simulink model "modelSim_QuanserAero_AdaptiveV3"  (R2025b)
settings: Solver=FixedStepAuto  StartTime=0.0  StopTime=T  FixedStep=DAQ_time  MaxStep=0.01  RelTol=1e-3
values from neighbouring files (symbols this model uses):
  A_cmd = [Ap_cmd, Ay_cmd]    [runExperiment_QuanserAero_Hardware_AdaptiveV4_1DOF_pitch.m]    (also in runExperiment_QuanserAero_Hardware_AdaptiveV4_1DOF_yaw.m; runSim_QuanserAero_AdaptiveV3.m; run_QuanserAero_AdaptiveV3_SN.m)
  a_cmd_coeff = [ap_cmd_coeff,ay_cmd_coeff]    [runExperiment_QuanserAero_Hardware_AdaptiveV4_1DOF_pitch.m]    (also in runExperiment_QuanserAero_Hardware_AdaptiveV4_1DOF_yaw.m; runSim_QuanserAero_AdaptiveV3.m; run_QuanserAero_AdaptiveV3_SN.m)
  cmd_select = [1,0]    [runExperiment_QuanserAero_Hardware_AdaptiveV4_1DOF_pitch.m]    (also in runExperiment_QuanserAero_Hardware_AdaptiveV4_1DOF_yaw.m = [1,1]; runSim_QuanserAero_AdaptiveV3.m = [0,2]; run_QuanserAero_AdaptiveV3_SN.m = [0,2])
  control_gains = [lambda_p lambda_y ... (first row only)    [runExperiment_QuanserAero_Hardware_AdaptiveV4_1DOF_pitch.m]    (also in runExperiment_QuanserAero_Hardware_AdaptiveV4_1DOF_yaw.m; runSim_QuanserAero_AdaptiveV3.m; run_QuanserAero_AdaptiveV3_SN.m)
  gamma_p = [gamma0_p;gamma1_p;gamma2_p;gamma3_p;gamma4_p]    [runExperiment_QuanserAero_Hardware_AdaptiveV4_1DOF_pitch.m]    (also in runExperiment_QuanserAero_Hardware_AdaptiveV4_1DOF_yaw.m; runSim_QuanserAero_AdaptiveV3.m; run_QuanserAero_AdaptiveV3_SN.m)
  gamma_y = [gamma0_y;gamma1_y;gamma2_y;gamma3_y]    [runExperiment_QuanserAero_Hardware_AdaptiveV4_1DOF_pitch.m]    (also in runExperiment_QuanserAero_Hardware_AdaptiveV4_1DOF_yaw.m; runSim_QuanserAero_AdaptiveV3.m; run_QuanserAero_AdaptiveV3_SN.m)
  harmonic_cutoff_p = Tp_cmd*harmonic_cycles    (= 20)    [runExperiment_QuanserAero_Hardware_AdaptiveV4_1DOF_pitch.m]    (also in runExperiment_QuanserAero_Hardware_AdaptiveV4_1DOF_yaw.m; runSim_QuanserAero_AdaptiveV3.m; run_QuanserAero_AdaptiveV3_SN.m)
  harmonic_cutoff_y = Ty_cmd*harmonic_cycles    (= 20)    [runExperiment_QuanserAero_Hardware_AdaptiveV4_1DOF_pitch.m]    (also in runExperiment_QuanserAero_Hardware_AdaptiveV4_1DOF_yaw.m; runSim_QuanserAero_AdaptiveV3.m; run_QuanserAero_AdaptiveV3_SN.m = 40)
  paramsGuess_haaaa = [hp_hat hy_hat ... (first row only)    [runExperiment_QuanserAero_Hardware_AdaptiveV4_1DOF_pitch.m]    (also in runExperiment_QuanserAero_Hardware_AdaptiveV4_1DOF_yaw.m; runSim_QuanserAero_AdaptiveV3.m; run_QuanserAero_AdaptiveV3_SN.m)
  paramsTruth_haaaa = paramsGuess_haaaa.*paramsError_haaaa    [runSim_QuanserAero_AdaptiveV3.m]    (also in run_QuanserAero_AdaptiveV3_SN.m)
  T_cmd = [Tp_cmd, Ty_cmd]    [runExperiment_QuanserAero_Hardware_AdaptiveV4_1DOF_pitch.m]    (also in runExperiment_QuanserAero_Hardware_AdaptiveV4_1DOF_yaw.m; runSim_QuanserAero_AdaptiveV3.m; run_QuanserAero_AdaptiveV3_SN.m)
settings Model: Creator=ryanmathewson  LastModifiedBy=samue
settings DebuggingCC: UnconnectedInputMsg=warning  UnconnectedOutputMsg=warning  UnconnectedLineMsg=warning
settings ModelReferenceCC: EnableRefExpFcnMdlSchedulingChecks=on
settings RTWCC: GPUComputeCapability=3.5  DLArmComputeVersion=19.05

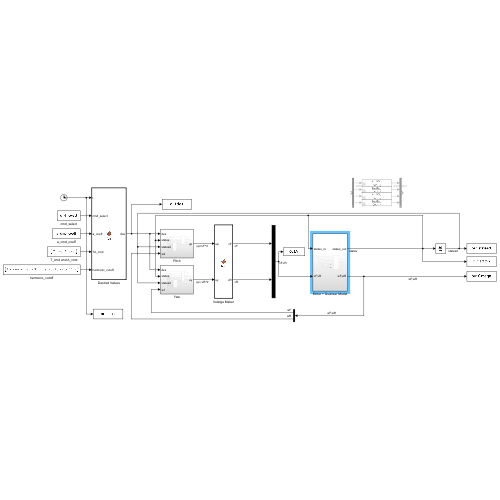
[thumbnail: Simulink's stored preview of the top-level diagram]
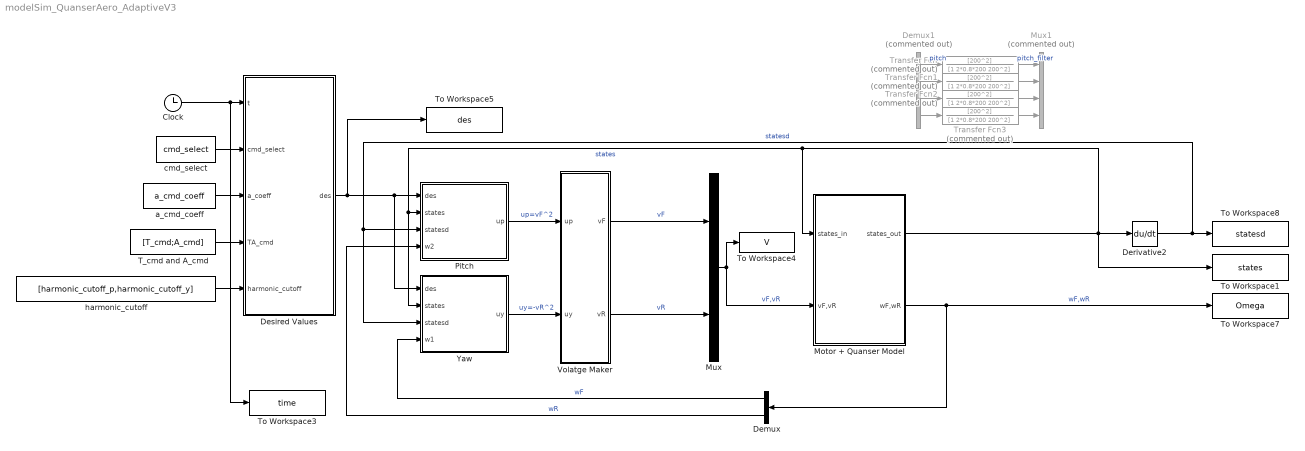
== system modelSim_QuanserAero_AdaptiveV3 ==
  Clock : Clock
  Demux : Demux  Outputs=2
  Demux1 : Demux  Commented=on
  Derivative2 : Derivative
  Desired Values : MATLAB Function  TreatAsAtomicUnit=on
  Motor + Quanser Model : Subsystem
  Mux : Mux  Inputs=2
  Mux1 : Mux  Commented=on
  Pitch : Subsystem
  T_cmd and A_cmd : Constant  Value=[T_cmd;A_cmd]
  To Workspace1 : ToWorkspace  VariableName=states  SampleTime=-1
  To Workspace3 : ToWorkspace  VariableName=time  SampleTime=-1
  To Workspace4 : ToWorkspace  VariableName=V  SampleTime=-1
  To Workspace5 : ToWorkspace  VariableName=des  SampleTime=-1
  To Workspace7 : ToWorkspace  VariableName=Omega  SampleTime=-1
  To Workspace8 : ToWorkspace  VariableName=statesd  SampleTime=-1
  Transfer Fcn{,1..3} (4 alike) : TransferFcn  Commented=on  Numerator=[200^2]  Denominator=[1 2*0.8*200 200^2]
  Volatge Maker : MATLAB Function  TreatAsAtomicUnit=on
  Yaw : Subsystem
  a_cmd_coeff : Constant  Value=a_cmd_coeff
  cmd_select : Constant  Value=cmd_select
  harmonic_cutoff : Constant  Value=[harmonic_cutoff_p,harmonic_cutoff_y]
  wires:
  Clock/1 -> To Workspace3/1, Desired Values/1(t)
  Desired Values/1(des) -> To Workspace5/1, Yaw/1(des), Pitch/1(des)
  Pitch/1(up) -> Volatge Maker/1(up)  "up=vF^2"
  Yaw/1(uy) -> Volatge Maker/2(uy)  "uy=-vR^2"
  Volatge Maker/1(vF) -> Mux/1  "vF"
  Derivative2/1 -> To Workspace8/1, Pitch/3(statesd), Yaw/3(statesd)  "statesd"
  Mux/1 -> Motor + Quanser Model/2(vF,vR), To Workspace4/1  "vF,vR"
  Volatge Maker/2(vR) -> Mux/2  "vR"
  Motor + Quanser Model/2(wF,wR) -> Demux/1, To Workspace7/1  "wF,wR"
  Demux/1 -> Yaw/4(w1)  "wF"
  Demux/2 -> Pitch/4(w2)  "wR"
  Motor + Quanser Model/1(states_out) -> Motor + Quanser Model/1(states_in), Pitch/2(states), Yaw/2(states), To Workspace1/1, Derivative2/1  "states"
  a_cmd_coeff/1 -> Desired Values/3(a_coeff)
  cmd_select/1 -> Desired Values/2(cmd_select)
  T_cmd and A_cmd/1 -> Desired Values/4(TA_cmd)
  harmonic_cutoff/1 -> Desired Values/5(harmonic_cutoff)
  Demux1/1 -> Transfer Fcn/1  "pitch"
  Demux1/3 -> Transfer Fcn2/1
  Demux1/2 -> Transfer Fcn1/1
  Demux1/4 -> Transfer Fcn3/1
  Transfer Fcn/1 -> Mux1/1  "pitch_filter"
  Transfer Fcn1/1 -> Mux1/2
  Transfer Fcn2/1 -> Mux1/3
  Transfer Fcn3/1 -> Mux1/4

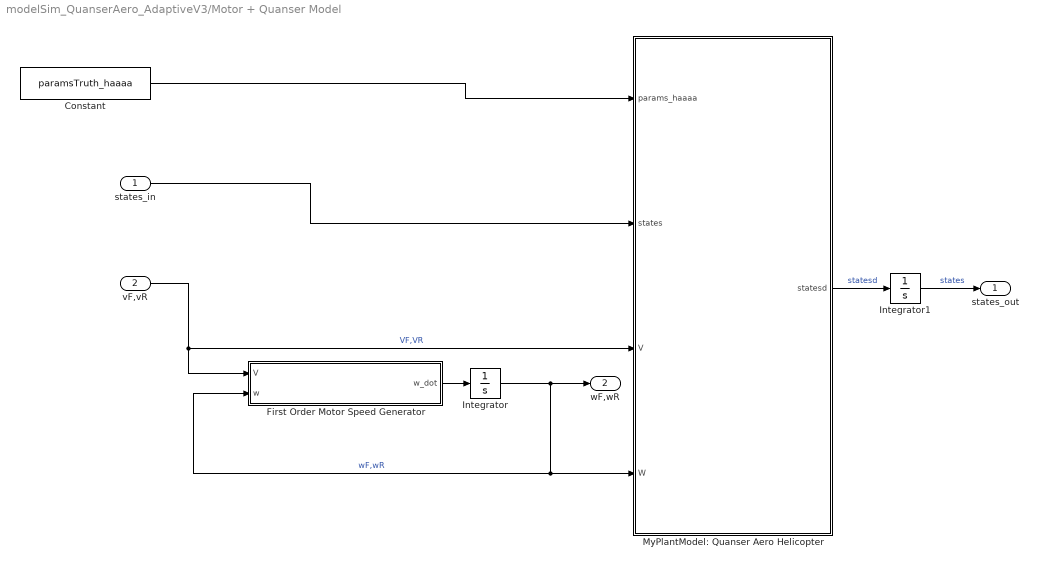
== system modelSim_QuanserAero_AdaptiveV3/Motor + Quanser Model ==
  states_in : Inport  PortDimensions=[4 1]
  vF,vR : Inport  Port=2  PortDimensions=[2 1]
  Constant : Constant  Value=paramsTruth_haaaa
  First Order Motor Speed Generator : MATLAB Function  TreatAsAtomicUnit=on
  Integrator : Integrator  InitialCondition=[0;0]
  Integrator1 : Integrator  InitialCondition=[0;0;0;0]
  MyPlantModel: Quanser Aero Helicopter : MATLAB Function  TreatAsAtomicUnit=on
  states_out : Outport  PortDimensions=[4 1]
  wF,wR : Outport  Port=2  PortDimensions=[2 1]
  wires:
  states_in/1 -> MyPlantModel: Quanser Aero Helicopter/2(states)
  vF,vR/1 -> First Order Motor Speed Generator/1(V), MyPlantModel: Quanser Aero Helicopter/3(V)  "VF,VR"
  MyPlantModel: Quanser Aero Helicopter/1(statesd) -> Integrator1/1  "statesd"
  First Order Motor Speed Generator/1(w_dot) -> Integrator/1
  Constant/1 -> MyPlantModel: Quanser Aero Helicopter/1(params_haaaa)
  Integrator1/1 -> states_out/1  "states"
  Integrator/1 -> First Order Motor Speed Generator/2(w), MyPlantModel: Quanser Aero Helicopter/4(W), wF,wR/1  "wF,wR"

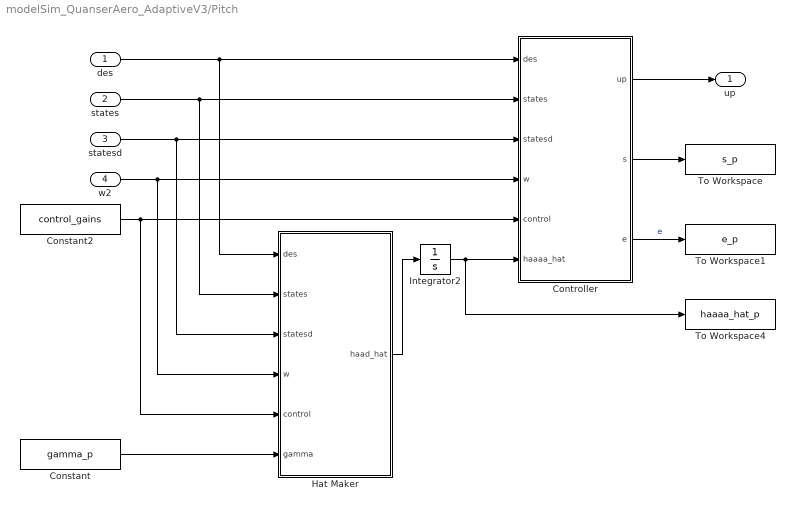
== system modelSim_QuanserAero_AdaptiveV3/Pitch ==
  des : Inport
  states : Inport  Port=2
  statesd : Inport  Port=3
  w2 : Inport  Port=4
  Constant : Constant  Value=gamma_p
  Constant2 : Constant  Value=control_gains
  Controller : MATLAB Function  TreatAsAtomicUnit=on
  Hat Maker : MATLAB Function  TreatAsAtomicUnit=on
  Integrator2 : Integrator  InitialCondition=paramsGuess_haaaa(:,1)
  To Workspace : ToWorkspace  VariableName=s_p  SampleTime=-1
  To Workspace1 : ToWorkspace  VariableName=e_p  SampleTime=-1
  To Workspace4 : ToWorkspace  VariableName=haaaa_hat_p  SampleTime=-1
  up : Outport
  wires:
  Integrator2/1 -> To Workspace4/1, Controller/6(haaaa_hat)
  Hat Maker/1(haad_hat) -> Integrator2/1
  Controller/1(up) -> up/1
  states/1 -> Hat Maker/2(states), Controller/2(states)
  Controller/2(s) -> To Workspace/1
  des/1 -> Hat Maker/1(des), Controller/1(des)
  statesd/1 -> Hat Maker/3(statesd), Controller/3(statesd)
  w2/1 -> Hat Maker/4(w), Controller/4(w)
  Constant2/1 -> Hat Maker/5(control), Controller/5(control)
  Constant/1 -> Hat Maker/6(gamma)
  Controller/3(e) -> To Workspace1/1  "e"

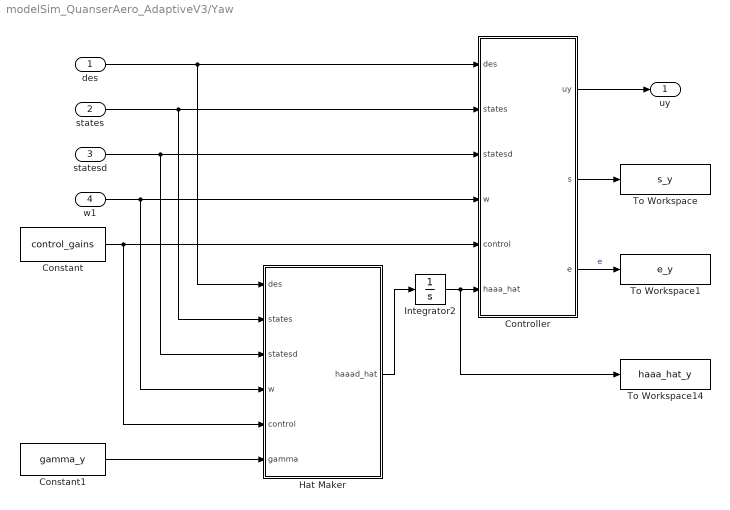
== system modelSim_QuanserAero_AdaptiveV3/Yaw ==
  des : Inport
  states : Inport  Port=2
  statesd : Inport  Port=3
  w1 : Inport  Port=4
  Constant : Constant  Value=control_gains
  Constant1 : Constant  Value=gamma_y
  Controller : MATLAB Function  TreatAsAtomicUnit=on
  Hat Maker : MATLAB Function  TreatAsAtomicUnit=on
  Integrator2 : Integrator  InitialCondition=paramsGuess_haaaa(1:4,2)
  To Workspace : ToWorkspace  VariableName=s_y  SampleTime=-1
  To Workspace1 : ToWorkspace  VariableName=e_y  SampleTime=-1
  To Workspace14 : ToWorkspace  VariableName=haaa_hat_y  SampleTime=-1
  uy : Outport
  wires:
  Integrator2/1 -> To Workspace14/1, Controller/6(haaa_hat)
  des/1 -> Controller/1(des), Hat Maker/1(des)
  Hat Maker/1(haaad_hat) -> Integrator2/1
  Controller/1(uy) -> uy/1
  Controller/2(s) -> To Workspace/1
  states/1 -> Controller/2(states), Hat Maker/2(states)
  statesd/1 -> Controller/3(statesd), Hat Maker/3(statesd)
  w1/1 -> Controller/4(w), Hat Maker/4(w)
  Controller/3(e) -> To Workspace1/1  "e"
  Constant/1 -> Controller/5(control), Hat Maker/5(control)
  Constant1/1 -> Hat Maker/6(gamma)

== matlab function modelSim_QuanserAero_AdaptiveV3/Yaw/Hat Maker ==
  data: des input; states input; haaad_hat output; statesd input; w input; control input; gamma input
function haaad_hat = fcn(des,states,statesd, w, control, gamma)
%% initialize outputs
haaad_hat = zeros(4,1);

%% separate input vectors
% desired variables
yaw_des = des(4,1);
yawd_des = des(5,1);
yawdd_des = des(6,1);
% state variables
r_yaw = states(3,1);
% state derivative variables
rd_yaw = statesd(3,1);
rdd_yaw = statesd(4,1);
% motor angular velocity
r_omega_f = w;
% controller gains
lambda = control(1,2);
D = control(2,2);
eta = control(3,2);
phi_para = control(4,2);
gamma_0 = gamma(1,1);
gamma_1 = gamma(2,1);
gamma_2 = gamma(3,1);
gamma_3 = gamma(4,1);

%% functions
e = r_yaw-yaw_des;
ed = rd_yaw-yawd_des;
yawdd_ref = -(-yawdd_des + lambda*ed) ; %2*lambda*ed + lambda^2*e;
s = ed + lambda*e;
ds = rdd_yaw - yawdd_ref;

%saturation function
% if s>phi_para
%   sat = 1;
% elseif (s>=-phi_para)&&(s<=phi_para)
%   sat = s/phi_para;
% else
%   sat = -1;
% end
if abs(s)>phi_para
    sat = sign(s);
else
    sat = s/phi_para;
end
s_delta = s - (phi_para * sat);

f1 = rd_yaw;
f2 = r_omega_f;
f3 = sign(r_omega_f)*r_omega_f^2;

%% outputs
hd_hat  = gamma_0^2 * s_delta * (yawdd_ref + ((D + eta) * sat));
a1d_hat = -gamma_1^2 * s_delta * f1;
a2d_hat = -gamma_2^2 * s_delta * f2;
a3d_hat = -gamma_3^2 * s_delta * f3;
haaad_hat = [hd_hat;a1d_hat;a2d_hat;a3d_hat];

== matlab function modelSim_QuanserAero_AdaptiveV3/Motor + Quanser Model/First Order Motor Speed Generator ==
  data: V input; w_dot output; w input
function w_dot = fcn(V, w)
% initialize output
w_dot = zeros(2,1);

% seperate input variables
V_f = V(1,1);
V_r = V(2,1);

w_f = w(1,1);
w_r = w(2,1);

% motor parameters
kt = 0.042219; % [N*m/A]
km = 0.042219; % [V/(rad/s)]
kd_f = 2.5e-7*abs(w_f) + 4.77e-06; % [N*m/(rad/s)]
kd_r = 2.5e-7*abs(w_r) + 4.77e-06; % [N*m/(rad/s)]
Rm = 8.4; % [Ohms]
Jm = 4e-6; % [kg*m^2]
Jh = 2.0160e-8; % [kg*m^2]
Jp = 4.0366e-5; % [kg*m^2]
Jeq = Jm+Jh+Jp; % [kg*m^2]

w_fdot = -(kt*km/(Rm*Jeq)+kd_f/Jeq)*w_f + (kt/(Rm*Jeq))*V_f;
w_rdot = -(kt*km/(Rm*Jeq)+kd_r/Jeq)*w_r + (kt/(Rm*Jeq))*V_r;

w_dot = [w_fdot;w_rdot];

== matlab function modelSim_QuanserAero_AdaptiveV3/Motor + Quanser Model/MyPlantModel: Quanser Aero Helicopter ==
  data: params_haaaa input; states input; V input; W input; statesd output
function statesd  = fcn(params_haaaa, states, V, W)
%% initialize output
statesd = zeros(4,1);
fn_p = zeros(4,1);
fn_y = zeros(3,1);

%% seperate voltage cmd
v_fc = V(1,1);
v_rc = V(2,1);

%% seperate states
w_fs = W(1,1);
w_rs = W(2,1);
pitch = states(1,1);
pitch_dot = states(2,1);
yaw = states(3,1);
yaw_dot = states(4,1);


%% model parameters
hp = params_haaaa(1,1);
ap1 = params_haaaa(2,1);
ap2 = params_haaaa(3,1);
ap3 = params_haaaa(4,1);
ap4 = params_haaaa(5,1);

hy =  params_haaaa(1,2);
ay1 = params_haaaa(2,2);
ay2 = params_haaaa(3,2);
ay3 = params_haaaa(4,2);

fp1 = pitch_dot;
fp2 = sin(pitch);
fp3 = w_rs;
fp4 = sign(w_rs)*w_rs^2;

fy1 = yaw_dot;
fy2 = w_fs;
fy3 = sign(w_fs)*w_fs^2;

%% Quanser Aero model
pitch_dotdot = -ap1/hp*fp1 -ap2/hp*fp2 -ap3/hp*fp3 -ap4/hp*fp4 ...
                              + 1/hp*sign(v_fc)*v_fc^2;

yaw_dotdot = -ay1/hy*fy1 -ay2/hy*fy2 -ay3/hy*fy3 ...
                              - 1/hy*sign(v_rc)*v_rc^2;

statesd = [pitch_dot;
           pitch_dotdot;
           yaw_dot
           yaw_dotdot];

fn_p = [fp1;fp2;fp3;fp4];
fn_y = [fy1;fy2;fy3];

== matlab function modelSim_QuanserAero_AdaptiveV3/Desired Values ==
  data: t input; des output; cmd_select input; a_coeff input; TA_cmd input; harmonic_cutoff input
function des = fcn(t,cmd_select,a_coeff,TA_cmd,harmonic_cutoff)
%% initialize outputs
des = zeros(6,1);

%% input parameters
ap_coeff = a_coeff(:,1); % polynomial coefficients for smooth step function
ay_coeff = a_coeff(:,2); % polynomial coefficients for smooth step function
Tp = TA_cmd(1,1); % pitch command period
Ty = TA_cmd(1,2); % yaw command period
PitchMag = TA_cmd(2,1); % pitch command amplitude
YawMag = TA_cmd(2,2); % yaw command amplitude
step_cos = cmd_select(1); % smooth step input or harmonic oscilator input selection
py_on_off = cmd_select(2); % pitch and yaw on or off selection
harmonic_cutoff_p = harmonic_cutoff(1); % time to command zero position, velocity, acceleration
harmonic_cutoff_y = harmonic_cutoff(2); % time to command zero position, velocity, acceleration

%% functions
if py_on_off == 0
    if step_cos == 0
        if t <= Tp
            pitch_des = ap_coeff(1)*t^4 + ap_coeff(2)*t^5 + ap_coeff(3)*t^6 + ap_coeff(4)*t^7;
            pitchd_des = 4*ap_coeff(1)*t^3 + 5*ap_coeff(2)*t^4 + 6*ap_coeff(3)*t^5 + 7*ap_coeff(4)*t^6;
            pitchdd_des = 12*ap_coeff(1)*t^2 + 20*ap_coeff(2)*t^3 + 30*ap_coeff(3)*t^4 + 42*ap_coeff(4)*t^5;
        else
            pitch_des = PitchMag;
            pitchd_des = 0;
            pitchdd_des = 0;
        end
        yaw_des = 0;
        yawd_des = 0;
        yawdd_des = 0;
    elseif step_cos == 1 && t<harmonic_cutoff_p
        pitch_des = (PitchMag/2)*(1-cos(2*pi*t/Tp));
        pitchd_des = (2*pi/Tp)*(PitchMag/2)*sin(2*pi*t/Tp);
        pitchdd_des = (2*pi/Tp)^2*(PitchMag/2)*cos(2*pi*t/Tp);
        yaw_des = 0;
        yawd_des = 0;
        yawdd_des = 0;
    elseif step_cos == 1 && t>=harmonic_cutoff_p
        pitch_des = 0;
        pitchd_des = 0;
        pitchdd_des = 0;
        yaw_des = 0;
        yawd_des = 0;
        yawdd_des = 0;
    else
        error("Not A Valid cmd_select")
    end
elseif py_on_off == 1
    if step_cos == 0
        pitch_des =0;
        pitchd_des = 0;
        pitchdd_des = 0;
        if t <= Ty
            yaw_des = ay_coeff(1)*t^4 + ay_coeff(2)*t^5 + ay_coeff(3)*t^6 + ay_coeff(4)*t^7;
            yawd_des = 4*ay_coeff(1)*t^3 + 5*ay_coeff(2)*t^4 + 6*ay_coeff(3)*t^5 + 7*ay_coeff(4)*t^6;
            yawdd_des = 12*ay_coeff(1)*t^2 + 20*ay_coeff(2)*t^3 + 30*ay_coeff(3)*t^4 + 42*ay_coeff(4)*t^5;
        else
            yaw_des = YawMag;
            yawd_des = 0;
            yawdd_des = 0;
        end
    elseif step_cos == 1 && t<harmonic_cutoff_y
        pitch_des =0;
        pitchd_des = 0;
        pitchdd_des = 0;
        yaw_des = (YawMag/2)*(1-cos(2*pi*t/Ty));
        yawd_des = (2*pi/Ty)*(YawMag/2)*sin(2*pi*t/Ty);
        yawdd_des = (2*pi/Ty)^2*(YawMag/2)*cos(2*pi*t/Ty);
    elseif step_cos == 1 && t>=harmonic_cutoff_y
        pitch_des =0;
        pitchd_des = 0;
        pitchdd_des = 0;
        yaw_des = 0;
        yawd_des = 0;
        yawdd_des = 0;
    else
        error("Not A Valid cmd_select")
    end
elseif py_on_off == 2
    if step_cos == 0
        if t <= Tp
            pitch_des = ap_coeff(1)*t^4 + ap_coeff(2)*t^5 + ap_coeff(3)*t^6 + ap_coeff(4)*t^7;
            pitchd_des = 4*ap_coeff(1)*t^3 + 5*ap_coeff(2)*t^4 + 6*ap_coeff(3)*t^5 + 7*ap_coeff(4)*t^6;
            pitchdd_des = 12*ap_coeff(1)*t^2 + 20*ap_coeff(2)*t^3 + 30*ap_coeff(3)*t^4 + 42*ap_coeff(4)*t^5;
        else
            pitch_des = PitchMag;
            pitchd_des = 0;
            pitchdd_des = 0;
        end
        if t <= Ty
            yaw_des = ay_coeff(1)*t^4 + ay_coeff(2)*t^5 + ay_coeff(3)*t^6 + ay_coeff(4)*t^7;
            yawd_des = 4*ay_coeff(1)*t^3 + 5*ay_coeff(2)*t^4 + 6*ay_coeff(3)*t^5 + 7*ay_coeff(4)*t^6;
            yawdd_des = 12*ay_coeff(1)*t^2 + 20*ay_coeff(2)*t^3 + 30*ay_coeff(3)*t^4 + 42*ay_coeff(4)*t^5;
        else
            yaw_des = YawMag;
            yawd_des = 0;
            yawdd_des = 0;
        end
    elseif  step_cos == 1
        if t<harmonic_cutoff_p
            pitch_des = (PitchMag/2)*(1-cos(2*pi*t/Tp));
            pitchd_des = (2*pi/Tp)*(PitchMag/2)*sin(2*pi*t/Tp);
            pitchdd_des = (2*pi/Tp)^2*(PitchMag/2)*cos(2*pi*t/Tp);
        else
            pitch_des = 0;
            pitchd_des = 0;
            pitchdd_des = 0;
        end
        if t<harmonic_cutoff_p
            yaw_des = (YawMag/2)*(1-cos(2*pi*t/Ty));
            yawd_des = (2*pi/Ty)*(YawMag/2)*sin(2*pi*t/Ty);
            yawdd_des = (2*pi/Ty)^2*(YawMag/2)*cos(2*pi*t/Ty);
        else
            yaw_des = 0;
            yawd_des = 0;
            yawdd_des = 0;
        end
    else
        error("Not A Valid cmd_select")
    end
else
    error("Not A Valid cmd_select")
end

des = [pitch_des;
       pitchd_des;
       pitchdd_des
       yaw_des;
       yawd_des;
       yawdd_des];

== matlab function modelSim_QuanserAero_AdaptiveV3/Volatge Maker ==
  data: vF output; vR output; up input; uy input
function [vF,vR] = fcn(up,uy)
% convert controller ouput to plant input (voltage)
vF = sqrt(abs(up))*sign(up);
vR = -sqrt(abs(uy))*sign(uy);

== matlab function modelSim_QuanserAero_AdaptiveV3/Pitch/Controller ==
  data: des input; states input; statesd input; w input; control input; up output; haaaa_hat input; s output; e output
function [up,s,e]= fcn(des,states,statesd,w,control,haaaa_hat)
%% initialize outputs
up = zeros(1,1);
s = zeros(1,1);
e = zeros(1,1);

%% separate input vectors
% desired variables
r_pitch_des = des(1,1);
rd_pitch_des = des(2,1);
rdd_pitch_des = des(3,1);
% state variables
r_pitch = states(1,1);
% state derivative variables
rd_pitch = statesd(1,1);
% motor angular speed
r_omega_r = w;
% controller gains
lambda = control(1,1);
D = control(2,1);
eta = control(3,1);
phi_para = control(4,1);
% estimated parameters
h_hat = haaaa_hat(1,1);
a1_hat = haaaa_hat(2,1);
a2_hat = haaaa_hat(3,1);
a3_hat = haaaa_hat(4,1);
a4_hat = haaaa_hat(5,1);

%% functions
e = r_pitch-r_pitch_des;
ed = rd_pitch-rd_pitch_des;
rdd_pitch_ref = rdd_pitch_des - lambda*ed; %+ 2*lambda*ed + lambda^2*e;
s = ed + lambda*e;

if abs(s)>phi_para
    sat = sign(s);
else
    sat = s/phi_para;
end

f1 = rd_pitch;
f2 = sin(r_pitch);
f3 = r_omega_r;
f4 = sign(r_omega_r)*r_omega_r^2;

%% outputs
up = - h_hat*(D+eta)*sat + h_hat*rdd_pitch_ref + a1_hat*f1 + a2_hat*f2 ...
                                              + a3_hat*f3 + a4_hat*f4;

== matlab function modelSim_QuanserAero_AdaptiveV3/Pitch/Hat Maker ==
  data: des input; states input; haad_hat output; statesd input; w input; control input; gamma input
function haad_hat = fcn(des,states,statesd,w,control,gamma)
%% initialize outputs
haad_hat = zeros(5,1);

%% separate input vectors
% desired variables
r_pitch_des = des(1,1);
rd_pitch_des = des(2,1);
rdd_pitch_des = des(3,1);
% state variables
r_pitch = states(1,1);
% state derivative variables
rd_pitch = statesd(1,1);
% motor angular speed
r_omega_r = w;
% controller gains
lambda = control(1,1);
D = control(2,1);
eta = control(3,1);
phi_para = control(4,1);
gamma_0 = gamma(1,1);
gamma_1 = gamma(2,1);
gamma_2 = gamma(3,1);
gamma_3 = gamma(4,1);
gamma_4 = gamma(5,1);

%% functions
e = r_pitch-r_pitch_des;
ed = rd_pitch-rd_pitch_des;
rdd_pitch_ref = -(-rdd_pitch_des + lambda*ed); %+ 2*lambda*ed + lambda^2*e;
s = ed + lambda*e;

if abs(s)>phi_para
    sat = sign(s);
else
    sat = s/phi_para;
end
s_delta = s - (phi_para * sat);

f1 = rd_pitch;
f2 = sin(r_pitch);
f3 = r_omega_r;
f4 = sign(r_omega_r)*r_omega_r^2;

%% outputs
hd_hat  = gamma_0^2 * s_delta * (rdd_pitch_ref + ((D + eta) * sat));
a1d_hat = -gamma_1^2 * s_delta * f1;
a2d_hat = -gamma_2^2 * s_delta * f2;
a3d_hat = -gamma_3^2 * s_delta * f3;
a4d_hat = -gamma_4^2 * s_delta * f4;
haad_hat = [hd_hat;
            a1d_hat;
            a2d_hat;
            a3d_hat;
            a4d_hat];

== matlab function modelSim_QuanserAero_AdaptiveV3/Yaw/Controller ==
  data: des input; states input; statesd input; w input; control input; uy output; haaa_hat input; s output; e output
function [uy,s,e]= fcn(des,states,statesd,w,control,haaa_hat)
%% initialize outputs
uy = zeros(1,1);
s = zeros(1,1);
e = zeros(1,1);

%% separate input vectors
% desired variables
yaw_des = des(4,1);
yawd_des = des(5,1);
yawdd_des = des(6,1);
% state variables
r_yaw = states(3,1);
% state derivative variables
rd_yaw = statesd(3,1);
% motor angular speed
r_omega_f = w;
% controller gains
lambda = control(1,2);
D = control(2,2);
eta = control(3,2);
phi_para = control(4,2);
% parameter estimations
h_hat = haaa_hat(1,1);
a1_hat = haaa_hat(2,1);
a2_hat = haaa_hat(3,1);
a3_hat = haaa_hat(4,1);

%% functions
e = r_yaw-yaw_des;
ed = rd_yaw-yawd_des;
yawdd_ref = yawdd_des - lambda*ed;
s = ed + lambda*e;

if abs(s)>phi_para
    sat = sign(s);
else
    sat = s/phi_para;
end

f1 = rd_yaw;
f2 = r_omega_f;
f3 = sign(r_omega_f)*r_omega_f^2;

%% outputs
uy = - h_hat*(D+eta)*sat + h_hat*yawdd_ref + a1_hat*f1 + a2_hat*f2 ...
                                                      + a3_hat*f3;
